simulink model "ArmRobot_function"  (R2020b)
settings: Solver=ode4  StartTime=0.0  StopTime=10.0  FixedStep=0.01  RelTol=1e-3
libraries: fuzblock x1
settings Model: Creator=Long  LastModifiedBy=Long

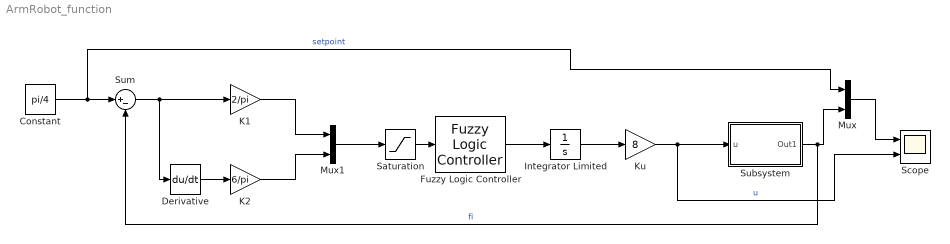
== system ArmRobot_function ==
  Constant : Constant  Value=pi/4
  Derivative : Derivative
  Fuzzy Logic Controller : fuzblock/Fuzzy Logic  Controller  FIS='ArmRobot_FuzzyController.fis'  OutputSampleNumber=101  DataType=double  FuzzifiedInputs=off  RuleFiringStrengths=off  RuleOutputs=off  AggregatedOutputs=off  SimulateUsing=Interpreted execution  OutOfRangeInputValueMessage=warning  NoRuleFiredMessage=warning  EmptyOutputFuzzySetMessage=warning
  Integrator Limited : Integrator  LimitOutput=on  UpperSaturationLimit=1  LowerSaturationLimit=-1
  K1 : Gain  Gain=2/pi
  K2 : Gain  Gain=6/pi
  Ku : Gain  Gain=8
  Mux : Mux  Inputs=2
  Mux1 : Mux  Inputs=2
  Saturation : Saturate  UpperLimit=1  LowerLimit=-1
  Scope : Scope  NumInputPorts=2
  Subsystem : Subsystem
  Sum : Sum  Inputs=|+-
  wires:
  Saturation/1 -> Fuzzy Logic Controller/1
  K1/1 -> Mux1/1
  K2/1 -> Mux1/2
  Derivative/1 -> K2/1
  Sum/1 -> Derivative/1, K1/1
  Constant/1 -> Mux/1, Sum/1  "setpoint"
  Mux1/1 -> Saturation/1
  Fuzzy Logic Controller/1 -> Integrator Limited/1
  Integrator Limited/1 -> Ku/1
  Ku/1 -> Scope/2, Subsystem/1(u)  "u"
  Subsystem/1(Out1) -> Mux/2, Sum/2  "fi"
  Mux/1 -> Scope/1

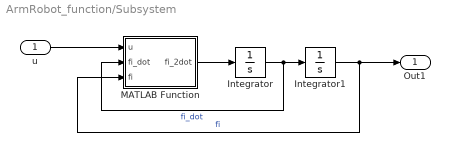
== system ArmRobot_function/Subsystem ==
  u : Inport
  Integrator : Integrator
  Integrator1 : Integrator
  MATLAB Function : MATLAB Function  TreatAsAtomicUnit=on
  Out1 : Outport
  wires:
  Integrator1/1 -> Out1/1, MATLAB Function/3(fi)  "fi"
  Integrator/1 -> MATLAB Function/2(fi_dot), Integrator1/1  "fi_dot"
  u/1 -> MATLAB Function/1(u)
  MATLAB Function/1(fi_2dot) -> Integrator/1

== matlab function ArmRobot_function/Subsystem/MATLAB Function ==
  data: u input; fi_2dot output; fi_dot input; fi input
function fi_2dot = fcn(u,fi_dot,fi)
J = 0.05;
M = 1;
l = 0.4;
lc = 0.15;
B = 0.2;
g = 9.81;
m = 0.1;
fi_2dot = (u-B*fi_dot-(m*l+M*lc)*g*sin(fi))/(J+m*l^2);
